simulink library "component_lib"  (R2023a)
settings: Solver=VariableStepAuto  StartTime=0.0  StopTime=10.0  RelTol=1e-3
undefined symbols (not defined in the file or in its folder): ECCV_r, par, R1234yf_ph, V_nom
libraries: base_lib x258, $bdroot x212, simulink x2, slpidlib x1
(part 2 of 7)

== system component_lib/Gas Exchange ==
  GE0001_humidGasSupply : Subsystem  mask{p_tot=1.01e5, x_H2=0, x_O2=0.21, RH=0, T=300}
      mask prompts: p_tot "Pressure [Pa]:"; x_H2 "Mole fraction dry H2 [-]:"; x_O2 "Mole fraction dry O2 [-]:"; RH "Relative humidity [-]:"; T "Temperature [K]:"
      mask init:
      | % parameter struct
      | par = struct;
      | 
      | par.p_tot = p_tot;
      | par.x_H2  = x_H2;
      | par.x_O2  = x_O2;
      | par.RH    = RH;
      | par.T     = T;
      | 
      | % par.p_tot = eval(get_param(gcb, 'p_tot'));
      | % par.x_H2  = eval(get_param(gcb, 'x_H2'));
      | % par.x_O2  = eval(get_param(gcb, 'x_O2'));
      | % par.RH    = eval(get_param(gcb, 'RH'));
      | % par.T     = eval(get_param(gcb, 'T'));
      | 
      | 
      | 
      | % Fixed parameters
      | par.R     = 8.314;  % [J/(mol*K)] - universal gas constant
      | par.M_N2  = 0.028;  % [kg/mol] - nitrogen molecular weight
      | par.M_H2O = 0.018;  % [kg/mol] - water
  GE0002_dynHumidGasSupply : Subsystem  mask{x_H2_dry=0, x_O2_dry=0.21}
      mask prompts: x_H2_dry "Mole-fraction dry hydrogen [-]:"; x_O2_dry "Mole-fraction dry oxygen [-]:"
      mask init:
      | % parameter struct
      | par = struct;
      | 
      | % Fixed parameters
      | par.R     = 8.314; % [J/(mol*K)] - universal gas constant
      | par.M_N2  = 0.028; % [kg/mol] - nitrogen molecular weight
      | par.M_H2O = 0.018; % [kg/mol] - water
  GE0007_hydrogenTank : Subsystem  mask{V=200e-3, T_tank=300, p_out=1.2e5, init_SOC=0.9, m0=5}
      mask prompts: V "Volume [m3]:"; T_tank "Tank temperature [K]:"; p_out "Outlet pressure [Pa]"; init_SOC "Initial charge [-]"; m0 "Total capacity [kg]:"
      mask init:
      | % parameter struct
      | par = struct;
      | 
      | % Get user-specified parameters
      | % par.V        = eval(get_param(gcb, 'V'));
      | % par.T_tank   = eval(get_param(gcb, 'T_tank'));
      | % par.p_out    = eval(get_param(gcb, 'p_out'));
      | % par.init_SOC = eval(get_param(gcb, 'init_SOC'));
      | % par.m0       = eval(get_param(gcb, 'm0'));
      | 
      | par.V        = V;
      | par.T_tank   = T_tank;
      | par.p_out    = p_out;
      | par.init_SOC = init_SOC;
      | par.m0       = m0;
      | 
      | 
      | % Standard state values
      | par.T0 = 298.15;  % [K]     - standard state temperature
      | par.h0 = 7.9260e3; % [J/mol] - standard state enthalpy
      | 
      | % Molar mass - [kg/mol]
      | par.M_j  = [0.002;
      |             0.032;
      |             0.018;
      |             0.028];    
      | 
      | % Specific heat - [J/kg*K]        
      | par.cp_j = [14.43e3;
      |             0.928e3;
      |             1.996e3;
      |             1.041e3];  
      | 
      | % Universal gas constant - [J/(mol*K)]   
      | par.R  = 8.314;         
      | 
      | % Specific gas constant [J/kg*K]
      | par.R_j = par.R ./ par.M_j;
  GE0008_gasProperties : Subsystem
  GE0009_controlVolume : Subsystem  mask{V=1.5833e-05, p0=1.01e5, x0_H2=0, x0_O2=0.21, RH0=0}
      mask prompts: V "Volume [m3]:"; p0 "Pressure [Pa]:"; x0_H2 "Mole fraction dry H2 [-]:"; x0_O2 "Mole fraction dry O2 [-]:"; RH0 "Relative humidity [-]:"
      mask init:
      | % parameter struct
      | par = struct;
      | 
      | % Get user-specified parameters
      | % par.V   = eval(get_param(gcb, 'V'));
      | par.V = V;
      | 
      | % initial conditions
      | par.p0    = p0;
      | par.x0_H2 = x0_H2;
      | par.x0_O2 = x0_O2;
      | par.RH0   = RH0;
      | 
      | % Molar mass - [kg/mol]
      | par.M_j  = [0.002;
      |             0.032;
      |             0.018;
      |             0.028];    
      | 
      | % Specific heat - [J/kg*K]        
      | par.cp_j = [14.43e3;
      |             0.928e3;
      |             1.996e3;
      |             1.041e3];  
      | 
      | % Universal gas constant - [J/(mol*K)]   
      | par.R  = 8.314;         
      | 
      | % Specific gas constant [J/kg*K]
      | par.R_j = par.R ./ par.M_j;
      mask DialogControl Container3 Prompt: Initial conditions:
  GE0010_compressibleRestriction : Subsystem  mask{C_d=1, D_t=1.84e-3, Pi_lin=0.97}
      mask prompts: C_d "Discharge coefficient [-]:"; D_t "Throat diameter [m]:"; Pi_lin "Lin. region  [-]"
      mask init:
      | % Check side
      | par = struct;
      | 
      | % parameters
      | par.C_d     = C_d;
      | par.Pi_lin  = Pi_lin;
      | par.D_t     = D_t;
      | 
      | % Molar mass - [kg/mol]
      | par.M_j  = [0.002;
      |             0.032;
      |             0.018;
      |             0.028];    
      | 
      | % Specific heat - [J/kg*K]        
      | par.cp_j = [14.43e3;
      |             0.928e3;
      |             1.996e3;
      |             1.041e3];  
      | 
      | % Universal gas constant - [J/(mol*K)]   
      | par.R  = 8.314;         
      | 
      | % Specific gas constant [J/kg*K]
      | par.R_j = par.R ./ par.M_j;
  GE0011_ellipseCompressor : Subsystem  mask{compressor_parameters=param_TD04.mat, w0=3e3}
      mask prompts: compressor_parameters "Parameter set:"; w0 "Initial speed [rad/s]:"
      mask init:
      | % parameter struct
      | % par = struct;
      | 
      | 
      | 
      | % find compressor models
      | compressorMaps = dir(fullfile('models/F0011_ellipseCompressor','*.mat'));
      | compressorMaps = {compressorMaps.name};
      | 
      | % update popup_list
      | msk = Simulink.Mask.get(gcb);
      | msk.Parameters(1).TypeOptions = compressorMaps;
      | 
      | % set profile
      | % try
      |     load(msk.Parameters(1).Value);
      | % end
      | 
      | % Get user-specified parameters
      | % par.w0   = eval(get_param(gcb, 'w0'));
      | par.w0   = w0;
      | 
      | 
      | % % Compressor parameters
      | % par.C_Wch       = [0.791459084209095;0.278369840595707;2.56393896117876;1.42688664691882];
      | % par.C_PIch      = [0.0903657853262553;0.467638667413134;4.35616456423884]; 
      | % par.C_Wzs       = [0.851951915665070;2.98625689994966];
      | % par.C_PIzs      = [1.24697676678299;2.08506798865712];
      | % par.C_cur       = [2.08068646432419;4.30416619749832;5.84893356036723];
      | % par.Gamma_PIcs  = [0.500000000000000];
      | % par.C_s         = [1.47023010236244];
      | % par.C_b         = [1.806586538255675;-0.642454577867690];
      | % par.C_a         = [0.863755184943499;0.033339263835893;24.999999984802365];
      | % par.C_loss      = 0.009455201151738;
      | % par.T_ref       =  298;
      | % par.p_ref       = 100000;
      | % par.Nc_max_map  = 1.860592187500000e+05;
      | % par.Wc_max_map  = 0.252151000000000;
      | % par.PI_max_map  = 2.766539113153419;
      | % par.Delta_h_max = 1.738661132271557e+05;
      | % par.gamma_air   = 1.397693997445722;
      | % par.rho1        = 1.169072149521521;
      | % par.D_2         = 0.056300000000000;
      | % par.Cp_air      = 1.008800956523303e+03;
      | % par.alpha_kPiW0 = 1.645763320284325;
      | % par.J_c         = 1.730000000000000e-05;
      | % par.c_fric      = 1e-6;
      | 
      | 
      | % Molar mass - [kg/mol]
      | par.M_j  = [0.002;
      |             0.032;
      |             0.018;
      |             0.028];    
      | 
      | % Specific heat - [J/kg*K]        
      | par.cp_j = [14.43e3;
      |             0.928e3;
      |             1.996e3;
      |             1.041e3];  
      | 
      | % Universal gas constant - [J/(mol*K)]   
      | par.R  = 8.314;         
      | 
      | % Specific gas constant [J/kg*K]
      | par.R_j = par.R ./ par.M_j;
      mask TypeOptions compressor_parameters: param_EK10C0822.mat | param_EK10C1220.mat | param_EK40C2429.mat | param_EK40C3425.mat | param_EK40C4521.mat | param_TD04.mat
  GE0012_throttle : Subsystem  mask{a0=1.3229e-05, a1=9.4736e-05, a2=0.0029, Pi_lin=0.97}
      mask prompts: Pi_lin "Lin. region  [-]"
      mask init:
      | % Check side
      | par = struct;
      | 
      | % parameters
      | par.Pi_lin  = Pi_lin;
      | 
      | par.C_d = 1;
      | par.a0 = a0;
      | par.a1 = a1;
      | par.a2 = a2;
      | 
      | % Molar mass - [kg/mol]
      | par.M_j  = [0.002;
      |             0.032;
      |             0.018;
      |             0.028];    
      | 
      | % Specific heat - [J/kg*K]        
      | par.cp_j = [14.43e3;
      |             0.928e3;
      |             1.996e3;
      |             1.041e3];  
      | 
      | % Universal gas constant - [J/(mol*K)]   
      | par.R  = 8.314;         
      | 
      | % Specific gas constant [J/kg*K]
      | par.R_j = par.R ./ par.M_j;
  GE0013_ejector : Subsystem  mask{C_d=1, D_t=1.84e-3, Pi_lin=0.97, c_0=0.78406, c_1=-0.85801}
      mask prompts: C_d "Discharge coefficient [-]:"; D_t "Nozzle throat diameter [m]:"; Pi_lin "Linear region [-]:"; c_0 "c0"; c_1 "c1"
      mask init:
      | % parameter struct
      | par = struct;
      | 
      | % Get user-specified parameters
      | % par.C_d    = eval(get_param(gcb, 'C_d'));
      | % par.D_t    = eval(get_param(gcb, 'D_t'));
      | % par.Pi_lin = eval(get_param(gcb, 'Pi_lin'));
      | % par.c_0     = eval(get_param(gcb, 'c_0'));
      | % par.c_1     = eval(get_param(gcb, 'c_1'));
      | 
      | par.C_d    = C_d;
      | par.D_t    = D_t;
      | par.Pi_lin = Pi_lin;
      | par.c_0    = c_0;
      | par.c_1    = c_1;
      |  
      | % Molar mass - [kg/mol]
      | par.M_j  = [0.002;
      |             0.032;
      |             0.018;
      |             0.028];    
      | 
      | % Specific heat - [J/kg*K]        
      | par.cp_j = [14.43e3;
      |             0.928e3;
      |             1.996e3;
      |             1.041e3];  
      | 
      | % Universal gas constant - [J/(mol*K)]   
      | par.R  = 8.314;         
      | 
      | % Specific gas constant [J/kg*K]
      | par.R_j = par.R ./ par.M_j;
  GE0014_flowValve : Subsystem  mask{C_d=1, D_t=1.84e-3, Pi_lin=0.97}
      mask prompts: C_d "Discharge coefficient [-]:"; D_t "Throat diameter [m]:"; Pi_lin "Lin. region  [-]"
      mask init: same as component_lib/Gas Exchange/GE0010_compressibleRestriction
  GE0015_linearRestriction : Subsystem  mask{C_d=4.7083e-08}
      mask prompts: C_d "Discharge coefficient [-]:"
      mask init:
      | % Check side
      | par = struct;
      | 
      | % parameters
      | % par.C_d     = eval(get_param(gcb, 'C_d'));
      | % par.tan_par = eval(get_param(gcb, 'tan_par'));
      | 
      | par.C_d     = C_d;
      | 
      | % Molar mass - [kg/mol]
      | par.M_j  = [0.002;
      |             0.032;
      |             0.018;
      |             0.028];    
      | 
      | % Specific heat - [J/kg*K]        
      | par.cp_j = [14.43e3;
      |             0.928e3;
      |             1.996e3;
      |             1.041e3];  
      | 
      | % Universal gas constant - [J/(mol*K)]   
      | par.R  = 8.314;         
      | 
      | % Specific gas constant [J/kg*K]
      | par.R_j = par.R ./ par.M_j;
  GE0016_simpleCompressor : Subsystem  mask{eta=0.7}
      mask prompts: eta "Efficiency [-]:"
  GE0017_humidifier : Subsystem  mask{T_s=30, gain=1}
      mask prompts: T_s "Time constant [s]:"; gain "Gain [RH -> Flow]:"
      mask init:
      | % parameter struct
      | par = struct;
      | 
      | 
      | % Molar mass - [kg/mol]
      | par.M_j  = [0.002;
      |             0.032;
      |             0.018;
      |             0.028];    
      | 
      | % Specific heat - [J/kg*K]        
      | par.cp_j = [14.43e3;
      |             0.928e3;
      |             1.996e3;
      |             1.041e3];  
      | 
      | % Universal gas constant - [J/(mol*K)]   
      | par.R  = 8.314;         
      | 
      | % Specific gas constant [J/kg*K]
      | par.R_j = par.R ./ par.M_j;
  GE0018_condenser : Subsystem  mask{T_s=1, gain=1}
      mask prompts: T_s "Time constant [s]:"; gain "Gain [RH -> Flow]:"
      mask init: same as component_lib/Gas Exchange/GE0017_humidifier
  GE0019_expander : Subsystem
      mask init:
      | % parameter struct
      | par = struct;
      | 
      | 
      | % Molar mass - [kg/mol]
      | par.M_j  = [0.002;
      |             0.032;
      |             0.018;
      |             0.028];    
      | 
      | % Specific heat - [J/kg*K]        
      | par.cp_j = [14.43e3;
      |             0.928e3;
      |             1.996e3;
      |             1.041e3];  
      | 
      | % Universal gas constant - [J/(mol*K)]   
      | par.R  = 8.314;         
      | 
      | % Specific gas constant [J/kg*K]
      | par.R_j = par.R ./ par.M_j; 
      | 
      | % turbine diameter
      | par.D = 0.0520;
      | 
      | % turbine efficiency model parameters
      | par.y = [-7.5046; -0.0012145; 3.5165e-07; 26.021; 0.00014675;
      |         -5.8187e-07; -20.162; 0.0018509; 1.6108e-07];
  GE0020_compressor : Subsystem  mask{compressor_parameters=param_TD04.mat}
      mask prompts: compressor_parameters "Parameter set:"
      mask init:
      | % parameter struct
      | % parameter struct
      | % par = struct;
      | 
      | 
      | 
      | % find compressor models
      | compressorMaps = dir(fullfile('models/F0011_ellipseCompressor','*.mat'));
      | compressorMaps = {compressorMaps.name};
      | 
      | % update popup_list
      | msk = Simulink.Mask.get(gcb);
      | msk.Parameters(1).TypeOptions = compressorMaps;
      | 
      | % set profile
      | % try
      |     load(msk.Parameters(1).Value);
      | % end
      | 
      | % Get user-specified parameters
      | % par.w0   = eval(get_param(gcb, 'w0'));
      | % par.w0   = w0;
      | 
      | 
      | % % Compressor parameters
      | % par.C_Wch       = [0.791459084209095;0.278369840595707;2.56393896117876;1.42688664691882];
      | % par.C_PIch      = [0.0903657853262553;0.467638667413134;4.35616456423884]; 
      | % par.C_Wzs       = [0.851951915665070;2.98625689994966];
      | % par.C_PIzs      = [1.24697676678299;2.08506798865712];
      | % par.C_cur       = [2.08068646432419;4.30416619749832;5.84893356036723];
      | % par.Gamma_PIcs  = [0.500000000000000];
      | % par.C_s         = [1.47023010236244];
      | % par.C_b         = [1.806586538255675;-0.642454577867690];
      | % par.C_a         = [0.863755184943499;0.033339263835893;24.999999984802365];
      | % par.C_loss      = 0.009455201151738;
      | % par.T_ref       =  298;
      | % par.p_ref       = 100000;
      | % par.Nc_max_map  = 1.860592187500000e+05;
      | % par.Wc_max_map  = 0.252151000000000;
      | % par.PI_max_map  = 2.766539113153419;
      | % par.Delta_h_max = 1.738661132271557e+05;
      | % par.gamma_air   = 1.397693997445722;
      | % par.rho1        = 1.169072149521521;
      | % par.D_2         = 0.056300000000000;
      | % par.Cp_air      = 1.008800956523303e+03;
      | % par.alpha_kPiW0 = 1.645763320284325;
      | % par.J_c         = 1.730000000000000e-05;
      | % par.c_fric      = 1e-6;
      | 
      | 
      | % Molar mass - [kg/mol]
      | par.M_j  = [0.002;
      |             0.032;
      |             0.018;
      |             0.028];    
      | 
      | % Specific heat - [J/kg*K]        
      | par.cp_j = [14.43e3;
      |             0.928e3;
      |             1.996e3;
      |             1.041e3];  
      | 
      | % Universal gas constant - [J/(mol*K)]   
      | par.R  = 8.314;         
      | 
      | % Specific gas constant [J/kg*K]
      | par.R_j = par.R ./ par.M_j;
      mask TypeOptions compressor_parameters: param_EK10C0822.mat | param_EK10C1220.mat | param_EK40C2429.mat | param_EK40C3425.mat | param_EK40C4521.mat | param_TD04.mat

== system component_lib/Mission ==
  MN0001_profile : Subsystem  mask{profile=KoblenzTrier.mat, x0=0, N_lookahead=100}
      mask prompts: profile "Road profile:"; x0 "Starting distance [m]:"; N_lookahead "Lookahead horizon [-]:"
      mask init:
      | % find road profiles in folder
      | availableProfiles = dir(fullfile('road_profiles','*.mat'));
      | availableProfiles = {availableProfiles.name};
      | 
      | % update popup_list
      | msk = Simulink.Mask.get(gcb);
      | msk.Parameters(1).TypeOptions = availableProfiles;
      | 
      | % set profile
      | try
      |     load(profile);
      | end
      mask TypeOptions profile: Helsingborg_to_Odeshog.mat | Helsingborg_to_Stockholm.mat | KoblenzTrier.mat | Munchen.mat | Odeshog_Goteborg.mat | Odeshog_to_Stockholm.mat | Sodertalje_Norrkoping.mat | flat_road.mat | incline.mat
      mask Display:
      | try
      |     plot(ECCV_r.distance, ECCV_r.altitude)
      | end
  MN0002_ambient : Subsystem  mask{p_0=1.01e5, T_0=298, RH_0=0.2}
      mask prompts: p_0 "Sea-level pressure [Pa]:"; T_0 "Sea-level temperature [K]:"; RH_0 "Sea-level humidity [-]:"
      mask init:
      | % parameter struct
      | par = struct;
      | 
      | % initial conditions
      | % par.p_0 = eval(get_param(gcb, 'p_0'));
      | % par.T_0 = eval(get_param(gcb, 'T_0'));
      | 
      | par.p_0 = p_0;
      | par.T_0 = T_0;

== system component_lib/Power Distribution Unit ==
  I_load [A] : Inport
  V_bat [V] : Inport  Port=2
  V_fc [V] : Inport  Port=3
  d [-] : Inport  Port=4
  bf [-] : Inport  Port=5
  Add : Sum
  Buck Converter : $bdroot/Electrochemistry/EL0004_buckCCM  R=1e-3  C=1  L=1e-3  V_init=340
  DC Bus : $bdroot/Electrochemistry/EL0006_busDC  R=1e-2  C=1  L=1e-3  V_init=340
  Gain : Gain  Gain=1/R_bf
  Product : Product
  Product1 : Product
  SC0002_signalRead1 : $bdroot/Data & Control/SC0002_signalRead  SigName=burnOffPower
  SC0002_signalRead10 : $bdroot/Data & Control/SC0002_signalRead  SigName=burnOffCurrent
  SC0002_signalRead2 : $bdroot/Data & Control/SC0002_signalRead  SigName=loadCurrent
  SC0002_signalRead3 : $bdroot/Data & Control/SC0002_signalRead  SigName=busVoltage
  Saturation : Saturate  UpperLimit=1  LowerLimit=0  ZeroCross=off
  Sum : Sum  Inputs=++|
  Transfer Fcn : TransferFcn  Denominator=[0.01 1]
  V_bus [V] : Outport
  I_bat [A] : Outport  Port=2
  I_fc [A] : Outport  Port=3
  I_bf [A] : Outport  Port=4
  Q_gen [J/s] : Outport  Port=5
  wires:
  DC Bus/3 -> Buck Converter/2
  V_bat [V]/1 -> DC Bus/1
  d [-]/1 -> Buck Converter/3
  V_fc [V]/1 -> Buck Converter/1
  Buck Converter/2 -> I_fc [A]/1
  DC Bus/1 -> I_bat [A]/1
  DC Bus/2 -> SC0002_signalRead3/1, Product1/2, Product/2, V_bus [V]/1
  Buck Converter/1 -> DC Bus/3
  Buck Converter/3 -> Add/1
  bf [-]/1 -> Saturation/1
  Saturation/1 -> Product/1
  I_load [A]/1 -> SC0002_signalRead2/1, Sum/2
  Sum/1 -> DC Bus/2
  Product/1 -> Gain/1
  Gain/1 -> Transfer Fcn/1
  Transfer Fcn/1 -> I_bf [A]/1, Product1/1, Sum/1, SC0002_signalRead10/1
  Product1/1 -> [Q_bf], SC0002_signalRead1/1
  Add/1 -> Q_gen [J/s]/1
  [Q_bf] -> Add/2

== system component_lib/Powertrain ==
  PT0001_simpleVehicle : Subsystem  mask{m=10e3, r_w=0.5, A_f=10, C_d=0.5, rho_air=1.225, c_r0=0.0060, c_r1=2.3e-7, gain=600, v0=0, x0=0}
      mask prompts: m "Vehicle mass [kg]:"; r_w "Wheel radius [m]:"; A_f "area [m2]:"; C_d "Flow coefficient:"; rho_air "air density [kg/m3]:"; v0 "Initial speed [m/s]:"; x0 "Initial position [m]:"
      mask init:
      | % parameter struct
      | par = struct;
      | 
      | % Get user-defined parameters
      | par.m        = m;
      | par.r_w      = r_w;
      | par.A_f      = A_f;
      | par.C_d      = C_d;
      | par.rho_air  = rho_air;
      | par.c_r0     = c_r0;
      | par.c_r1     = c_r1;
      | par.gain     = gain;
      | par.v0       = v0;
      | par.x0       = x0;
      mask DialogControl ParameterGroupVar Prompt: General
      mask DialogControl Container5 Prompt: Air drag
      mask DialogControl Container4 Prompt: Rolling resistance
      mask DialogControl Container7 Prompt: Brake
      mask DialogControl Container3 Prompt: Initial conditions
  PT0002_simpleMotor : Subsystem  mask{T_s=0.1}
      mask prompts: T_s "Torque time cont. [s]:"
      mask init:
      | % parameter struct
      | par = struct;
      | 
      | % motor parameters
      | par.e  = 0.86692;
      | par.c1 = 319.3242;
      | par.c2 = -7.3604;
      | par.c3 = 0.060174;
  PT0003_gearBox : Subsystem  mask{fd_ratio=2, gear_ratios=[5 3.8 2.3 1.15], eta_gb=0.98}
      mask prompts: fd_ratio "Final drive ratio [-]:"; gear_ratios "Gear ratios [-]:"; eta_gb "Efficiency [-]:"
      mask init:
      | % parameters
      | par = struct;
      | 
      | par.fd_ratio    = fd_ratio;
      | par.gear_ratios = gear_ratios;
      | par.eta_gb      = eta_gb;
      | par.gears       = 1:length(par.gear_ratios);
  PT0004_electricMachine : Subsystem  mask{T_s=0.1}
      mask prompts: T_s "Torque time cont. [s]:"
      mask init:
      | % parameter struct
      | par = struct;
      | 
      | % motor parameters
      | par.e  = 0.86692;
      | par.c1 = 319.3242;
      | par.c2 = -7.3604;
      | par.c3 = 0.060174;

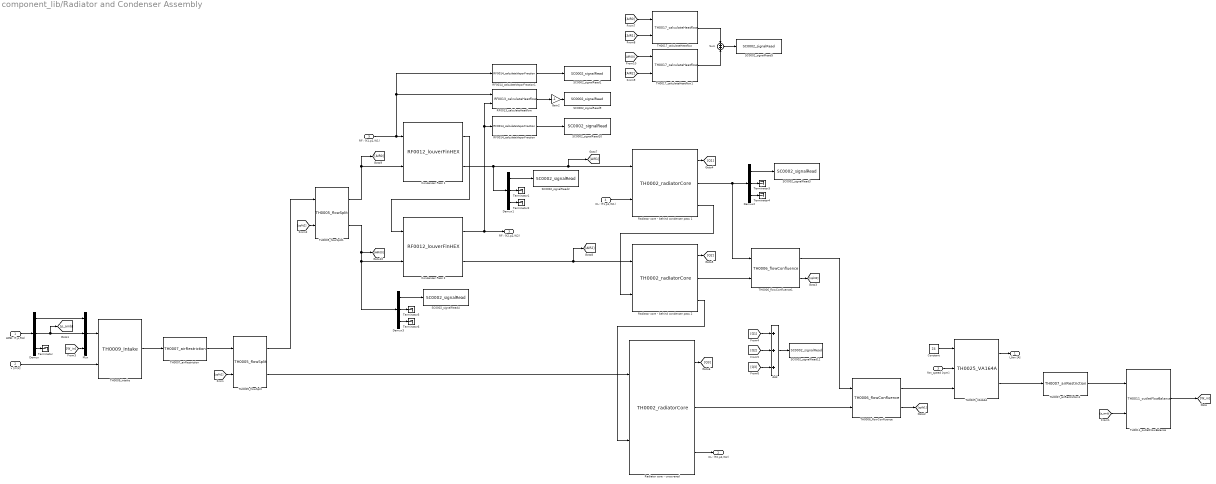
== system component_lib/Radiator and Condenser Assembly ==
  AMB: (T,p,RH) : Inport
  v [m/s] : Inport  Port=2
  fan_speed [rpm] : Inport  Port=3
  CL: (T1,p1,W1) : Inport  Port=4
  RF: (h1,p1,W1) : Inport  Port=5
  Add : Sum  Inputs=+++
  Condenser Pass 1 : $bdroot/Thermal Systems/RF0012_louverFinHEX  h00=400e3  N_tub=40  T_L=0.95  T_p=10.15e-3  T_d=16e-3  N_ch=18  a=1.3e-3  b=0.58e-3  L_a=23  F_p=1.4e-3  L_p=1.7e-3  L_l=6.4e-3  H=8.15e-3  d_f=16e-3  F_d=16e-3  N_nod=5
  Condenser Pass 2 : $bdroot/Thermal Systems/RF0012_louverFinHEX  h00=400e3  N_tub=40  T_L=0.95  T_p=10.15e-3  T_d=16e-3  N_ch=18  a=1.3e-3  b=0.58e-3  L_a=23  F_p=1.4e-3  L_p=1.7e-3  L_l=6.4e-3  H=8.15e-3  d_f=16e-3  F_d=16e-3  N_nod=5
  Constant : Constant  Value=24
  Demux{,1..3} (4 alike) : Demux  Outputs=3
  Gain2 : Gain  Gain=-1
  Mux : Mux  Inputs=3
  RF0013_calculateHeatflow : $bdroot/Thermal Systems/RF0013_calculateHeatflow
  RF0014_calculateVaporFraction : $bdroot/Thermal Systems/RF0014_calculateVaporFraction
  RF0014_calculateVaporFraction1 : $bdroot/Thermal Systems/RF0014_calculateVaporFraction
  Radiator core - behind condenser pass 1 : $bdroot/Thermal Systems/TH0002_radiatorCore  HtH=0.4060  StS=0.95  radmodel=52 mm
  Radiator core - behind condenser pass 2 : $bdroot/Thermal Systems/TH0002_radiatorCore  HtH=0.4060  StS=0.95  radmodel=52 mm
  Radiator core - uncovered : $bdroot/Thermal Systems/TH0002_radiatorCore  HtH=1.1- 2 * 0.4060  StS=0.95  radmodel=52 mm
  SC0002_signalRead1 : $bdroot/Data & Control/SC0002_signalRead  SigName=vaporFractionCondenserInlet
  SC0002_signalRead10 : $bdroot/Data & Control/SC0002_signalRead  SigName=vaporFractionCondenserOutlet
  SC0002_signalRead12 : $bdroot/Data & Control/SC0002_signalRead  SigName=radiatorCooling
  SC0002_signalRead2 : $bdroot/Data & Control/SC0002_signalRead  SigName=airTemperatureAfterCondenser
  SC0002_signalRead3 : $bdroot/Data & Control/SC0002_signalRead  SigName=airTemperatureAfterRadiator
  SC0002_signalRead4 : $bdroot/Data & Control/SC0002_signalRead  SigName=airTemperatureIntake
  SC0002_signalRead5 : $bdroot/Data & Control/SC0002_signalRead  SigName=condenserAirHeating
  SC0002_signalRead9 : $bdroot/Data & Control/SC0002_signalRead  SigName=condenserCooling
  Sum : Sum  Inputs=+|+
  TH0005_flowSplit : $bdroot/Thermal Systems/TH0005_flowSplit  SystemSampleTime=-1  VariantActivationTime=update diagram  Latency=0  AutoFrameSizeCalculation=off
  TH0005_flowSplit1 : $bdroot/Thermal Systems/TH0005_flowSplit  SystemSampleTime=-1  VariantActivationTime=update diagram  Latency=0  AutoFrameSizeCalculation=off
  TH0006_flowConfluence : $bdroot/Thermal Systems/TH0006_flowConfluence  gain=0.01
  TH0006_flowConfluence1 : $bdroot/Thermal Systems/TH0006_flowConfluence  gain=0.01
  TH0007_airRestriction : $bdroot/Thermal Systems/TH0007_airRestriction  A=0.8  zeta=0.3
  TH0007_airRestriction1 : $bdroot/Thermal Systems/TH0007_airRestriction  A=1  zeta=2.5
  TH0009_intake : $bdroot/Thermal Systems/TH0009_intake  zeta=0.9
  TH0011_outletFlowBalance : $bdroot/Thermal Systems/TH0011_outletFlowBalance  gain=0.05
  TH0017_calculateHeatflow : $bdroot/Thermal Systems/TH0017_calculateHeatflow
  TH0017_calculateHeatflow1 : $bdroot/Thermal Systems/TH0017_calculateHeatflow
  TH0025_VA164A : $bdroot/Thermal Systems/TH0025_VA164A  n=1
      settings: LibrarySourceBlock=component_lib/Thermal Systems/TH0023_WP120
  Terminator{,1..6} (7 alike) : Terminator
  I_fan [A] : Outport
  CL: (T2,p2,W2) : Outport  Port=2
  RF: (h2,p2,W2) : Outport  Port=3
  wires:
  Demux/2 -> Mux/2, [p_amb]
  Demux/1 -> Mux/1
  AMB: (T,p,RH)/1 -> Demux/1
  Radiator core - uncovered/3 -> CL: (T2,p2,W2)/1
  fan_speed [rpm]/1 -> TH0025_VA164A/2
  v [m/s]/1 -> TH0009_intake/2
  TH0007_airRestriction/1 -> TH0005_flowSplit/1
  TH0007_airRestriction1/1 -> TH0011_outletFlowBalance/1
  Mux/1 -> TH0009_intake/1
  TH0009_intake/1 -> TH0007_airRestriction/1
  Radiator core - uncovered/2 -> TH0006_flowConfluence/2
  [p_amb] -> TH0011_outletFlowBalance/2
  TH0005_flowSplit/2 -> Radiator core - uncovered/1
  TH0025_VA164A/2 -> TH0007_airRestriction1/1
  TH0011_outletFlowBalance/1 -> [W_in]
  [W_in] -> Mux/3
  Demux/3 -> Terminator/1
  CL: (T1,p1,W1)/1 -> Radiator core - behind condenser pass 1/2
  TH0005_flowSplit/1 -> TH0005_flowSplit1/1
  Condenser Pass 2/1 -> RF0013_calculateHeatflow/2, RF0014_calculateVaporFraction/1, RF: (h2,p2,W2)/1
  Condenser Pass 1/1 -> Condenser Pass 2/1
  Condenser Pass 1/2 -> [AIR1], Radiator core - behind condenser pass 1/1, Demux1/1
  Condenser Pass 2/2 -> [AIR2], Radiator core - behind condenser pass 2/1
  TH0005_flowSplit1/1 -> [AIR0], Condenser Pass 1/2
  Radiator core - behind condenser pass 1/3 -> Radiator core - behind condenser pass 2/2
  Radiator core - behind condenser pass 2/3 -> Radiator core - uncovered/2
  Radiator core - behind condenser pass 2/2 -> TH0006_flowConfluence1/2
  TH0006_flowConfluence1/1 -> TH0006_flowConfluence/1
  [split1] -> TH0005_flowSplit/2
  TH0006_flowConfluence/2 -> [split1]
  [split2] -> TH0005_flowSplit1/2
  TH0006_flowConfluence1/2 -> [split2]
  RF0013_calculateHeatflow/1 -> Gain2/1
  Gain2/1 -> SC0002_signalRead9/1
  Add/1 -> SC0002_signalRead12/1
  RF0014_calculateVaporFraction/1 -> SC0002_signalRead10/1
  RF0014_calculateVaporFraction1/1 -> SC0002_signalRead1/1
  RF: (h1,p1,W1)/1 -> RF0014_calculateVaporFraction1/1, RF0013_calculateHeatflow/1, Condenser Pass 1/1
  Radiator core - behind condenser pass 1/1 -> [Q1]
  Radiator core - behind condenser pass 2/1 -> [Q2]
  Radiator core - uncovered/1 -> [Q3]
  [Q1] -> Add/1
  [Q2] -> Add/2
  [Q3] -> Add/3
  Demux1/2 -> Terminator1/1
  Demux1/3 -> Terminator2/1
  Demux1/1 -> SC0002_signalRead2/1
  Radiator core - behind condenser pass 1/2 -> TH0006_flowConfluence1/1, Demux2/1
  Demux2/3 -> Terminator4/1
  Demux2/2 -> Terminator3/1
  Demux2/1 -> SC0002_signalRead3/1
  TH0005_flowSplit1/2 -> Demux3/1, Condenser Pass 2/2, [AIR00]
  Demux3/3 -> Terminator6/1
  Demux3/2 -> Terminator5/1
  Demux3/1 -> SC0002_signalRead4/1
  [AIR0] -> TH0017_calculateHeatflow/1
  [AIR1] -> TH0017_calculateHeatflow/2
  [AIR2] -> TH0017_calculateHeatflow1/2
  TH0017_calculateHeatflow/1 -> Sum/1
  TH0017_calculateHeatflow1/1 -> Sum/2
  Sum/1 -> SC0002_signalRead5/1
  [AIR00] -> TH0017_calculateHeatflow1/1
  TH0006_flowConfluence/1 -> TH0025_VA164A/3
  TH0025_VA164A/1 -> I_fan [A]/1
  Constant/1 -> TH0025_VA164A/1

== system component_lib/Simple Fuel Cell System ==
  I [A] : Inport
  T [K] : Inport  Port=2
  Constant : Constant  Value=2.5e5
  Constant1 : Constant  Value=0.8
  Constant2 : Constant  Value=2.5e5
  Constant3 : Constant  Value=0.8
  Constant4 : Constant  Value=n
  EL0007_pukrushpan2004 : $bdroot/Electrochemistry/EL0007_pukrushpan2004  U_0=1  j_0=1e-3  alpha=0.25  ASR=1e-1  A_fc=420
  F0010_vaporSaturationPressure.m : base_lib/F0010_gasFlow/F0010_vaporSaturationPressure.m  SystemSampleTime=-1  VariantActivationTime=update diagram  Latency=0  AutoFrameSizeCalculation=off
      settings: LibrarySourceBlock=|
      | simulink/User-Defined
      | Functions/MATLAB Function
  GE0002_dynHumidGasSupply : $bdroot/Gas Exchange/GE0002_dynHumidGasSupply  x_H2_dry=0  x_O2_dry=0.21
  GE0002_dynHumidGasSupply1 : $bdroot/Gas Exchange/GE0002_dynHumidGasSupply  x_H2_dry=1  x_O2_dry=0
  Gain : Gain  Gain=n_st
  Gain1 : Gain  Gain=n_st
  Gain2 : Gain  Gain=n_st
  Product{1..5} (5 alike) : Product
  SC0002_signalRead1 : $bdroot/Data & Control/SC0002_signalRead  SigName=fuelCellVoltage
  SC0002_signalRead3 : $bdroot/Data & Control/SC0002_signalRead  SigName=membraneWaterContent
  SC0002_signalRead4 : $bdroot/Data & Control/SC0002_signalRead  SigName=fuelCellPower
  SC0002_signalRead5 : $bdroot/Data & Control/SC0002_signalRead  SigName=vaporSaturationPressure
  SC0002_signalRead6 : $bdroot/Data & Control/SC0002_signalRead  SigName=singleCellVoltage
  SC0002_signalRead8 : $bdroot/Data & Control/SC0002_signalRead  SigName=fuelCellCurrent
  Subsystem1 : Subsystem
      mask Display: disp('Fuel consumption calculation [kg/100km]');
  V [V] : Outport
  Q_gen [J/s] : Outport  Port=2
  wires:
  Product1/1 -> Gain1/1
  Product2/1 -> [W_an], Gain/1
  Product5/1 -> [W_ca]
  Constant4/1 -> Product1/2, Product2/2, Product5/2, Product3/2
  EL0007_pukrushpan2004/3 -> Product5/1
  EL0007_pukrushpan2004/2 -> Product2/1
  EL0007_pukrushpan2004/5 -> Product3/1
  Product4/1 -> SC0002_signalRead4/1
  EL0007_pukrushpan2004/4 -> SC0002_signalRead3/1
  T [K]/1 -> F0010_vaporSaturationPressure.m/1, EL0007_pukrushpan2004/4, EL0007_pukrushpan2004/5, EL0007_pukrushpan2004/6, GE0002_dynHumidGasSupply1/1, GE0002_dynHumidGasSupply/1
  F0010_vaporSaturationPressure.m/1 -> SC0002_signalRead5/1
  Gain/1 -> Subsystem1/1(In1)
  Gain1/1 -> V [V]/1, SC0002_signalRead1/1, Product4/2
  Product3/1 -> Gain2/1
  Gain2/1 -> Q_gen [J/s]/1
  GE0002_dynHumidGasSupply1/1 -> EL0007_pukrushpan2004/2
  GE0002_dynHumidGasSupply/1 -> EL0007_pukrushpan2004/3
  I [A]/1 -> EL0007_pukrushpan2004/1, SC0002_signalRead8/1, Product4/1
  EL0007_pukrushpan2004/1 -> SC0002_signalRead6/1, Product1/1
  Constant/1 -> GE0002_dynHumidGasSupply/2
  Constant1/1 -> GE0002_dynHumidGasSupply/3
  Constant3/1 -> GE0002_dynHumidGasSupply1/3
  Constant2/1 -> GE0002_dynHumidGasSupply1/2

== system component_lib/Simple Fuel Cell System ITPEM ==
  I [A] : Inport
  T [K] : Inport  Port=2
  p_tot [Pa] : Inport  Port=3
  RH [-] : Inport  Port=4
  Constant4 : Constant  Value=n
  Demux : Demux
  EL0011_ITPEMFC : $bdroot/Electrochemistry/EL0011_ITPEMFC  A_fc=A_fc
  GE0002_dynHumidGasSupply : $bdroot/Gas Exchange/GE0002_dynHumidGasSupply  x_H2_dry=0  x_O2_dry=0.21
  Gain : Gain  Gain=n_st
  Gain1 : Gain  Gain=n_st
  Gain2 : Gain  Gain=n_st
  Product{1..5} (5 alike) : Product
  SC0002_signalRead1 : $bdroot/Data & Control/SC0002_signalRead  SigName=fuelCellVoltage
  SC0002_signalRead4 : $bdroot/Data & Control/SC0002_signalRead  SigName=fuelCellPower
  SC0002_signalRead8 : $bdroot/Data & Control/SC0002_signalRead  SigName=fuelCellCurrent
  Subsystem1 : Subsystem
      mask Display: disp('Fuel consumption calculation [kg/100km]');
  Terminator : Terminator
  Terminator1 : Terminator
  Terminator2 : Terminator
  V [V] : Outport
  Q_gen [J/s] : Outport  Port=2
  wires:
  Product1/1 -> Gain1/1
  Product2/1 -> Gain/1
  Product5/1 -> [W_ca]
  Constant4/1 -> Product3/2, Product5/2, Product2/2, Product1/2
  EL0011_ITPEMFC/4 -> Product3/1
  Product4/1 -> SC0002_signalRead4/1
  T [K]/1 -> GE0002_dynHumidGasSupply/1
  Gain/1 -> Subsystem1/1(In1)
  Gain1/1 -> V [V]/1, Product4/2, SC0002_signalRead1/1
  Product3/1 -> Gain2/1
  Gain2/1 -> Q_gen [J/s]/1
  I [A]/1 -> EL0011_ITPEMFC/1, Product4/1, SC0002_signalRead8/1
  EL0011_ITPEMFC/1 -> Product1/1
  p_tot [Pa]/1 -> GE0002_dynHumidGasSupply/2
  RH [-]/1 -> EL0011_ITPEMFC/4, GE0002_dynHumidGasSupply/3
  GE0002_dynHumidGasSupply/1 -> Demux/1
  Demux/2 -> EL0011_ITPEMFC/2
  Demux/1 -> Terminator/1
  Demux/3 -> Terminator1/1
  Demux/4 -> Terminator2/1
  EL0011_ITPEMFC/2 -> Product2/1
  EL0011_ITPEMFC/3 -> Product5/1
  GE0002_dynHumidGasSupply/2 -> EL0011_ITPEMFC/3

== system component_lib/Single Air Stream 3x Radiator ==
  AMB: (T,p,RH) : Inport
  v [m/s] : Inport  Port=2
  rel_fan_speed [-] : Inport  Port=3
  CL A: (T1,p1,W1) : Inport  Port=4
  CL B: (T1,p1,W1) : Inport  Port=5
  CL C: (T1,p1,W1) : Inport  Port=6
  Battery Circuit Radiator : $bdroot/Thermal Systems/TH0002_radiatorCore  HtH=1.1  StS=0.95  radmodel=52 mm
  Demux : Demux  Outputs=3
  Fuel Cell Circuit Radiator : $bdroot/Thermal Systems/TH0002_radiatorCore  HtH=1.1  StS=0.95  radmodel=52 mm
  Fuel Cell Circuit Radiator1 : $bdroot/Thermal Systems/TH0002_radiatorCore  HtH=1.1  StS=0.95  radmodel=52 mm
  Mux : Mux  Inputs=3
  TH0003_coolantTank{,1..5} (6 alike) : $bdroot/Thermal Systems/TH0003_coolantTank  StS=0.95  D_con=0.055  T_0=286  radmodel=52 mm
  TH0004_radiatorPlugFlow : $bdroot/Thermal Systems/TH0004_radiatorPlugFlow  HtH=1.1  StS=0.95  T_0=286  radmodel=52 mm
  TH0004_radiatorPlugFlow1 : $bdroot/Thermal Systems/TH0004_radiatorPlugFlow  HtH=1.1  StS=0.95  T_0=286  radmodel=52 mm
  TH0004_radiatorPlugFlow2 : $bdroot/Thermal Systems/TH0004_radiatorPlugFlow  HtH=1.1  StS=0.95  T_0=286  radmodel=52 mm
  TH0007_airRestriction : $bdroot/Thermal Systems/TH0007_airRestriction  A=0.8  zeta=0.3
  TH0007_airRestriction1 : $bdroot/Thermal Systems/TH0007_airRestriction  A=1  zeta=2.5
  TH0009_intake : $bdroot/Thermal Systems/TH0009_intake  zeta=0.9
  TH0010_fan : $bdroot/Thermal Systems/TH0010_fan  n_fan=10
  TH0011_outletFlowBalance : $bdroot/Thermal Systems/TH0011_outletFlowBalance  gain=0.05
  P_fan [J/s] : Outport
  CL A: (T2,p2,W2) : Outport  Port=2
  CL B: (T2,p2,W2) : Outport  Port=3
  CL C: (T2,p2,W2) : Outport  Port=4
  wires:
  Demux/2 -> Mux/2, [p_amb]
  Demux/1 -> Mux/1
  AMB: (T,p,RH)/1 -> Demux/1
  TH0003_coolantTank1/1 -> CL A: (T2,p2,W2)/1
  TH0010_fan/2 -> P_fan [J/s]/1
  rel_fan_speed [-]/1 -> TH0010_fan/2
  v [m/s]/1 -> TH0009_intake/2
  TH0004_radiatorPlugFlow/1 -> TH0003_coolantTank1/1
  TH0007_airRestriction1/1 -> TH0011_outletFlowBalance/1
  CL A: (T1,p1,W1)/1 -> TH0003_coolantTank/1
  Mux/1 -> TH0009_intake/1
  TH0009_intake/1 -> TH0007_airRestriction/1
  TH0003_coolantTank/1 -> Battery Circuit Radiator/2
  [p_amb] -> TH0011_outletFlowBalance/2
  TH0007_airRestriction/1 -> Battery Circuit Radiator/1
  TH0010_fan/1 -> TH0007_airRestriction1/1
  Battery Circuit Radiator/3 -> TH0004_radiatorPlugFlow/1
  TH0011_outletFlowBalance/1 -> [W_in]
  [W_in] -> Mux/3
  Battery Circuit Radiator/2 -> Fuel Cell Circuit Radiator/1
  Fuel Cell Circuit Radiator/2 -> Fuel Cell Circuit Radiator1/1
  TH0004_radiatorPlugFlow1/1 -> TH0003_coolantTank2/1
  TH0003_coolantTank2/1 -> CL B: (T2,p2,W2)/1
  Fuel Cell Circuit Radiator/3 -> TH0004_radiatorPlugFlow1/1
  Fuel Cell Circuit Radiator1/3 -> TH0004_radiatorPlugFlow2/1
  TH0003_coolantTank3/1 -> CL C: (T2,p2,W2)/1
  TH0004_radiatorPlugFlow2/1 -> TH0003_coolantTank3/1
  TH0003_coolantTank4/1 -> Fuel Cell Circuit Radiator/2
  CL B: (T1,p1,W1)/1 -> TH0003_coolantTank4/1
  TH0003_coolantTank5/1 -> Fuel Cell Circuit Radiator1/2
  CL C: (T1,p1,W1)/1 -> TH0003_coolantTank5/1
  Fuel Cell Circuit Radiator1/2 -> TH0010_fan/1

== system component_lib/Single Air Stream Heat Exchanger ==
  AMB: (T,p,RH) : Inport
  v [m/s] : Inport  Port=2
  fan_speed [rpm] : Inport  Port=3
  CL: (T1,p1,W1) : Inport  Port=4
  Constant : Constant  Value=24
  Demux : Demux  Outputs=3
  Mux : Mux  Inputs=3
  Radiator core - exposed : $bdroot/Thermal Systems/TH0002_radiatorCore  HtH=0.6  StS=0.6  radmodel=52 mm
  TH0003_coolantTank : $bdroot/Thermal Systems/TH0003_coolantTank  StS=0.95  D_con=0.055  T_0=286  radmodel=52 mm
  TH0003_coolantTank1 : $bdroot/Thermal Systems/TH0003_coolantTank  StS=0.95  D_con=0.055  T_0=286  radmodel=52 mm
  TH0004_radiatorPlugFlow : $bdroot/Thermal Systems/TH0004_radiatorPlugFlow  HtH=1.1  StS=0.95  T_0=286  radmodel=52 mm
  TH0007_airRestriction : $bdroot/Thermal Systems/TH0007_airRestriction  A=0.8  zeta=0.3
  TH0007_airRestriction1 : $bdroot/Thermal Systems/TH0007_airRestriction  A=1  zeta=2.5
  TH0009_intake : $bdroot/Thermal Systems/TH0009_intake  zeta=0.9
  TH0011_outletFlowBalance : $bdroot/Thermal Systems/TH0011_outletFlowBalance  gain=0.05
  TH0025_VA164A : $bdroot/Thermal Systems/TH0025_VA164A  n=1
      settings: LibrarySourceBlock=component_lib/Thermal Systems/TH0023_WP120
  I_fan [A] : Outport
  CL: (T2,p2,W2) : Outport  Port=2
  wires:
  Demux/2 -> Mux/2, [p_amb]
  Demux/1 -> Mux/1
  AMB: (T,p,RH)/1 -> Demux/1
  TH0003_coolantTank1/1 -> CL: (T2,p2,W2)/1
  TH0025_VA164A/1 -> I_fan [A]/1
  fan_speed [rpm]/1 -> TH0025_VA164A/2
  v [m/s]/1 -> TH0009_intake/2
  TH0004_radiatorPlugFlow/1 -> TH0003_coolantTank1/1
  TH0007_airRestriction1/1 -> TH0011_outletFlowBalance/1
  CL: (T1,p1,W1)/1 -> TH0003_coolantTank/1
  Mux/1 -> TH0009_intake/1
  TH0009_intake/1 -> TH0007_airRestriction/1
  TH0003_coolantTank/1 -> Radiator core - exposed/2
  [p_amb] -> TH0011_outletFlowBalance/2
  TH0007_airRestriction/1 -> Radiator core - exposed/1
  TH0025_VA164A/2 -> TH0007_airRestriction1/1
  Radiator core - exposed/3 -> TH0004_radiatorPlugFlow/1
  TH0011_outletFlowBalance/1 -> [W_in]
  [W_in] -> Mux/3
  Radiator core - exposed/2 -> TH0025_VA164A/3
  Constant/1 -> TH0025_VA164A/1

== system component_lib/Thermal Mass & Heat Transfer ==
  Q_in [J/s] : Inport
  CL: (T1,p1,W1) : Inport  Port=2
  Sum : Sum  Inputs=|+-
  TH0011_coolingChannel : $bdroot/Thermal Systems/TH0011_coolingChannel  d=d  L=L  n_ch=n  e=0.006e-3
  TH0011_thermalMass : $bdroot/Thermal Systems/TH0011_thermalMass  m=m  cp=cp  T_0=T_0
  T_ [K] : Outport
  CL: (T2,p2,W2) : Outport  Port=2
  wires:
  Sum/1 -> TH0011_thermalMass/1
  TH0011_thermalMass/1 -> T_ [K]/1, TH0011_coolingChannel/1
  TH0011_coolingChannel/1 -> Sum/2
  Q_in [J/s]/1 -> Sum/1
  CL: (T1,p1,W1)/1 -> TH0011_coolingChannel/2
  TH0011_coolingChannel/2 -> CL: (T2,p2,W2)/1
